simulink model "myQpskXmtSim"  (Simulink 7.7)
settings: Solver=ode45  StartTime=0.0  StopTime=1/fmod*1000  RelTol=1e-3
PreLoadFcn:
  | fcar = 1e9;
  | fmod = 10e6;
  | fs = fcar*10;
StopFcn:
  | [f,dataOut] = myFft(sigOut,fs,16,'MHz',1);
  | axis([(fcar-fmod*8)/1e6 (fcar+fmod*8)/1e6 -90 0]);
libraries: commrandsrc2 x2, dsparch4 x2, dspstat3 x1
settings Model: Creator=acarroll  LastModifiedBy=acarroll

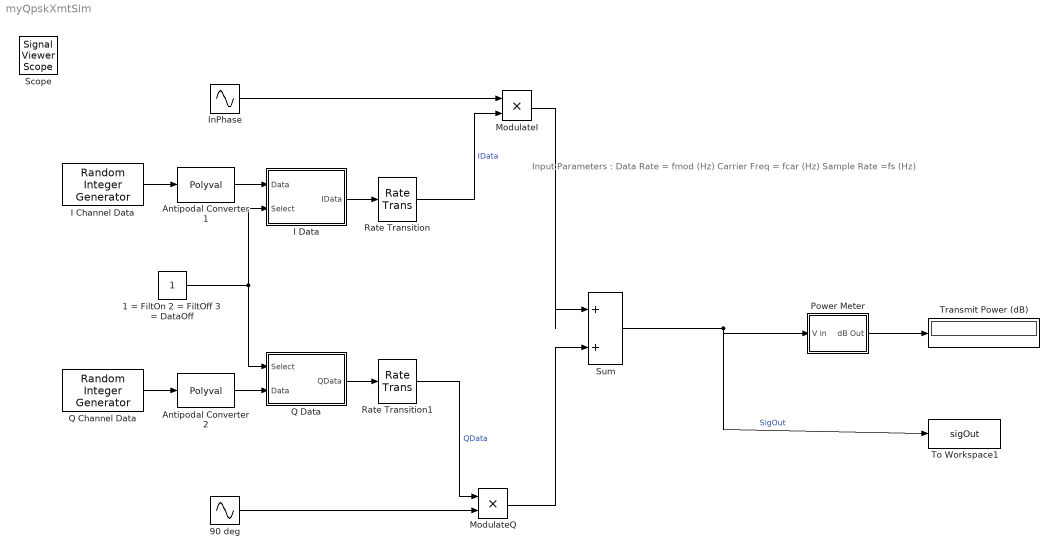
== system myQpskXmtSim ==
  note: Input Parameters :
      |     Data Rate  = fmod (Hz)
      |     Carrier Freq  = fcar (Hz)
      |     Sample Rate  =fs (Hz)
  1 = FiltOn 2 = FiltOff 3 = DataOff : Constant
  90 deg : Sin  SineType=Sample based  Samples=fs/fcar  SampleTime=1/fs  Offset=fs/fcar/4
  Antipodal Converter 1 : Polyval  Coefs=[ 2 -1 ]
  Antipodal Converter 2 : Polyval  Coefs=[ 2 -1 ]
  I Channel Data : commrandsrc2/Random Integer Generator  SystemSampleTime=-1  mul=2  seed=randseed  Ts=1/fmod  frameBased=off  sampPerFrame=50  orient=on  outDataType=double
  I Data : Subsystem
  InPhase : Sin  SineType=Sample based  Samples=fs/fcar  SampleTime=1/fs
  ModulateI : Product  RndMeth=Zero
  ModulateQ : Product  RndMeth=Zero
  "Power Meter " : Subsystem
  Q Channel Data : commrandsrc2/Random Integer Generator  SystemSampleTime=-1  mul=2  seed=randseed  Ts=1/fmod  frameBased=off  sampPerFrame=50  orient=on  outDataType=double
  Q Data : Subsystem
  Rate Transition : RateTransition  OutPortSampleTime=1/fs
  Rate Transition1 : RateTransition  OutPortSampleTime=1/fs
  Sum : Sum  Inputs=|++
  To Workspace1 : ToWorkspace  VariableName=sigOut  SampleTime=1/fs  SaveFormat=Array
  Transmit Power (dB) : Display
  Scope : SignalViewerScope  IOType=viewer  NumInputPorts=3  ZoomMode=xonly  RefreshTime=0.035000
      settings: YMin=-5~-5~-5  YMax=5~5~5  MaxDataPoints=750000
  wires:
  I Channel Data/1 -> Antipodal Converter 1/1
  "Power Meter "/1(dB Out) -> Transmit Power (dB)/1
  InPhase/1 -> ModulateI/1
  Q Channel Data/1 -> Antipodal Converter 2/1
  90 deg/1 -> ModulateQ/2
  ModulateI/1 -> Sum/1
  ModulateQ/1 -> Sum/2
  Sum/1 -> To Workspace1/1, "Power Meter "/1(V in)  "SigOut"
  Rate Transition/1 -> ModulateI/2  "IData"
  Rate Transition1/1 -> ModulateQ/1  "QData"
  Q Data/1(QData) -> Rate Transition1/1
  Antipodal Converter 2/1 -> Q Data/2(Data)
  I Data/1(IData) -> Rate Transition/1
  Antipodal Converter 1/1 -> I Data/1(Data)
  1 = FiltOn 2 = FiltOff 3 = DataOff/1 -> Q Data/1(Select), I Data/2(Select)

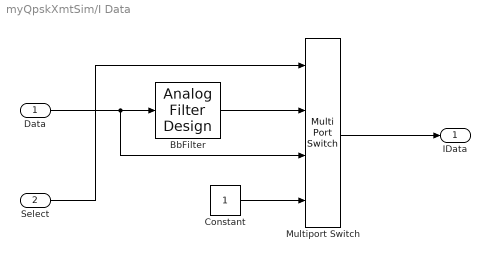
== system myQpskXmtSim/I Data ==
  Data : Inport
  Select : Inport  Port=2
  BbFilter : dsparch4/Analog Filter Design  method=Bessel  filttype=Lowpass  N=4  Wlo=2*pi*55e6  Whi=80  Rp=2  Rs=40
  Constant : Constant
  Multiport Switch : MultiPortSwitch  zeroidx=off
  IData : Outport
  wires:
  Data/1 -> BbFilter/1, Multiport Switch/3
  Multiport Switch/1 -> IData/1
  Constant/1 -> Multiport Switch/4
  BbFilter/1 -> Multiport Switch/2
  Select/1 -> Multiport Switch/1

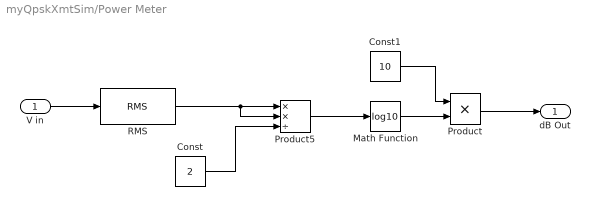
== system myQpskXmtSim/Power Meter  ==
  V in : Inport
  Const : Constant  Value=2
  Const1 : Constant  Value=10
  Math Function : Math  Operator=log10  SaturateOnIntegerOverflow=on
  Product : Product  RndMeth=Zero
  Product5 : Product  Inputs=**/  RndMeth=Zero
  RMS : dspstat3/RMS  run=on  reset_popup=None  InputProcessing=Inherited (this choice will be removed - see release notes)  directionMode=Each column  dimension=1  treatSBRowAsCol=on
  dB Out : Outport
  wires:
  Const/1 -> Product5/3
  RMS/1 -> Product5/2, Product5/1
  V in/1 -> RMS/1
  Product5/1 -> Math Function/1
  Math Function/1 -> Product/2
  Const1/1 -> Product/1
  Product/1 -> dB Out/1

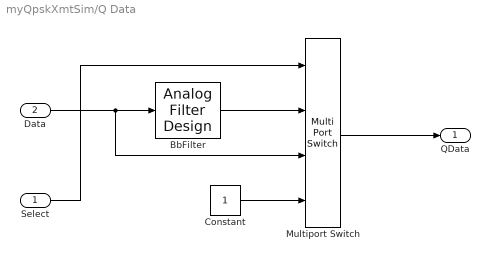
== system myQpskXmtSim/Q Data ==
  Select : Inport
  Data : Inport  Port=2
  BbFilter : dsparch4/Analog Filter Design  method=Bessel  filttype=Lowpass  N=4  Wlo=2*pi*55e6  Whi=80  Rp=2  Rs=40
  Constant : Constant
  Multiport Switch : MultiPortSwitch  zeroidx=off
  QData : Outport
  wires:
  Multiport Switch/1 -> QData/1
  Data/1 -> BbFilter/1, Multiport Switch/3
  Constant/1 -> Multiport Switch/4
  BbFilter/1 -> Multiport Switch/2
  Select/1 -> Multiport Switch/1
